simulink model "twist_filter_sl"  (R2018b)
settings: Solver=FixedStepDiscrete  StartTime=0.0  StopTime=inf  FixedStep=0.1  RelTol=1e-3
model workspace (MAT data in the model file):
  ERROR = 1e-08
undefined symbols (not defined in the file): Header, Twist
libraries: robotlib x5, simulink x1
settings Model: Creator=sdd  LastModifiedBy=sdd
settings DataIOCC: SaveOutput=off  SignalLogging=off  DSMLogging=off  SaveTime=off
settings OptimizationCC: EnhancedBackFolding=on  PassReuseOutputArgsThreshold=0  MaxStackSize=64  OptimizeBlockOrder=speed  DifferentSizesBufferReuse=on  OptimizationCustomize=off
settings DebuggingCC: ParameterTunabilityLossMsg=error  LibraryContextMissingDiagnostic=none
settings HardwareCC: ProdBitPerPointer=32  ProdBitPerSizeT=32  ProdBitPerPtrDiffT=32  ProdLargestAtomicFloat=None  ProdIntDivRoundTo=Undefined  ProdEndianess=Unspecified  ProdWordSize=32  ProdHWDeviceType=Generic->Unspecified (assume 32-bit Generic)  UseEmbeddedCoderFeatures=off
settings SFSimCC: SimUseLocalCustomCode=off  MATLABDynamicMemAlloc=off
settings RTWCC: SystemTargetFile=ert.tlc  HardwareBoard=Robot Operating System (ROS)  TLCOptions="-aInlineSetEventsForThisBaseRateFcn=TLC_FALSE -aSuppressMultiTaskScheduler=TLC_FALSE  -aRateBasedStepFcn=0"  TemplateMakefile=ert_default_tmf  GenerateReport=on  RTWUseLocalCustomCode=off  Toolchain=Catkin  LaunchReport=on  TargetLang=C++
settings CodeAppCC: ForceParamTrailComments=on  OperatorAnnotations=on
settings ERTTargetCC: ERTCustomFileBanners=off  SupportContinuousTime=on  SupportNonInlinedSFcns=on  RemoveResetFunc=off  ModelStepFunctionPrototypeControlCompliant=off

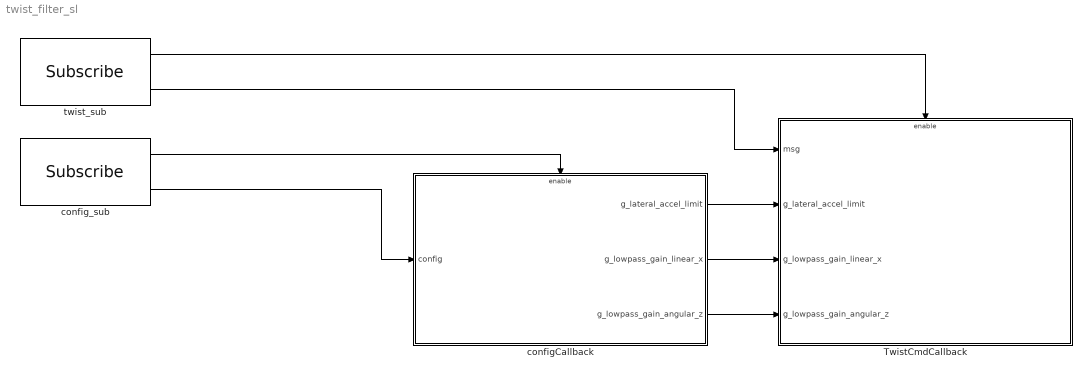
== system twist_filter_sl ==
  TwistCmdCallback : Subsystem
  configCallback : Subsystem
  config_sub : robotlib/Subscribe  topicSource=Select from ROS network  topic=/config/twist_filter  messageType=autoware_msgs/ConfigTwistFilter  sampleTime=-1  messageQueueLength=1
      settings: SourceProductBaseCode=RO
  twist_sub : robotlib/Subscribe  topicSource=Select from ROS network  topic=/twist_raw  messageType=geometry_msgs/TwistStamped  sampleTime=-1  messageQueueLength=1
      settings: SourceProductBaseCode=RO
  wires:
  configCallback/1(g_lateral_accel_limit) -> TwistCmdCallback/2(g_lateral_accel_limit)
  configCallback/2(g_lowpass_gain_linear_x) -> TwistCmdCallback/3(g_lowpass_gain_linear_x)
  configCallback/3(g_lowpass_gain_angular_z) -> TwistCmdCallback/4(g_lowpass_gain_angular_z)
  config_sub/1 -> configCallback/Enable
  config_sub/2 -> configCallback/1(config)
  twist_sub/1 -> TwistCmdCallback/Enable
  twist_sub/2 -> TwistCmdCallback/1(msg)

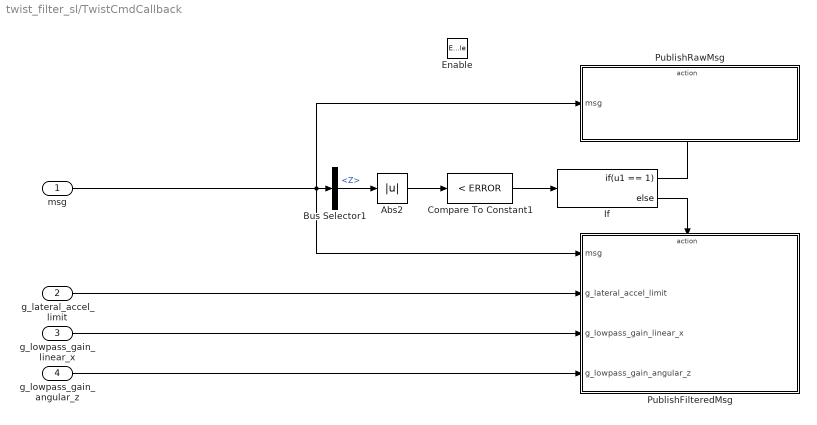
== system twist_filter_sl/TwistCmdCallback ==
  msg : Inport  Interpolate=off  BusOutputAsStruct=on
  g_lateral_accel_limit : Inport  Port=2
  g_lowpass_gain_linear_x : Inport  Port=3
  g_lowpass_gain_angular_z : Inport  Port=4
  Enable : EnablePort
  Abs2 : Abs
  Bus Selector1 : BusSelector  OutputSignals=Twist.Angular.Z
  Compare To Constant1 : simulink/Logic and Bit Operations/Compare To Constant  relop=<  const=ERROR  OutDataTypeStr=boolean
  If : If  IfExpression=u1 == 1
  PublishFilteredMsg : Subsystem
  PublishRawMsg : Subsystem  TreatAsAtomicUnit=on
  wires:
  g_lowpass_gain_angular_z/1 -> PublishFilteredMsg/4(g_lowpass_gain_angular_z)
  g_lowpass_gain_linear_x/1 -> PublishFilteredMsg/3(g_lowpass_gain_linear_x)
  Compare To Constant1/1 -> If/1
  If/2 -> PublishFilteredMsg/Action
  Bus Selector1/1 -> Abs2/1  "<Z>"
  msg/1 -> PublishFilteredMsg/1(msg), PublishRawMsg/1(msg), Bus Selector1/1
  Abs2/1 -> Compare To Constant1/1
  g_lateral_accel_limit/1 -> PublishFilteredMsg/2(g_lateral_accel_limit)
  If/1 -> PublishRawMsg/Action

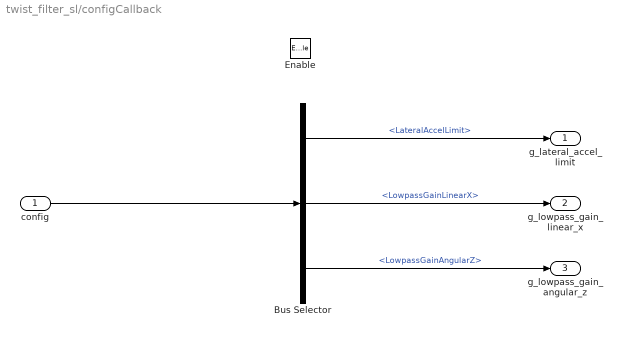
== system twist_filter_sl/configCallback ==
  config : Inport
  Enable : EnablePort
  Bus Selector : BusSelector  OutputSignals=LateralAccelLimit,LowpassGainLinearX,LowpassGainAngularZ
  g_lateral_accel_limit : Outport  InitialOutput=5
  g_lowpass_gain_linear_x : Outport  Port=2  InitialOutput=0
  g_lowpass_gain_angular_z : Outport  Port=3  InitialOutput=0
  wires:
  Bus Selector/3 -> g_lowpass_gain_angular_z/1  "<LowpassGainAngularZ>"
  Bus Selector/2 -> g_lowpass_gain_linear_x/1  "<LowpassGainLinearX>"
  config/1 -> Bus Selector/1
  Bus Selector/1 -> g_lateral_accel_limit/1  "<LateralAccelLimit>"

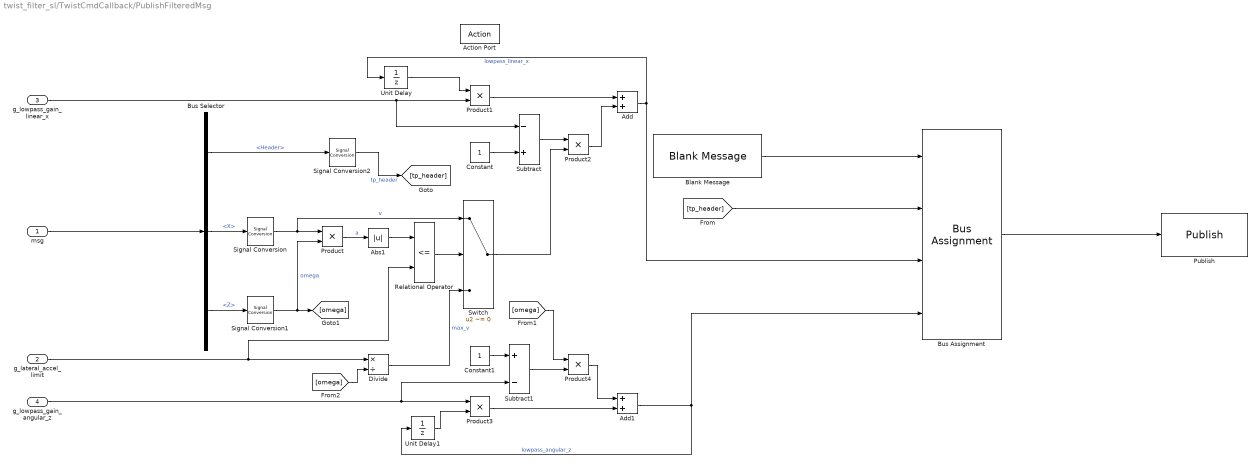
== system twist_filter_sl/TwistCmdCallback/PublishFilteredMsg ==
  msg : Inport
  g_lateral_accel_limit : Inport  Port=2
  g_lowpass_gain_linear_x : Inport  Port=3
  g_lowpass_gain_angular_z : Inport  Port=4
  Action Port : ActionPort  ActionType=else
  Abs1 : Abs
  Add : Sum
  Add1 : Sum
  Blank Message : robotlib/Blank Message  messageClass=Message  entityType=geometry_msgs/TwistStamped  messageType=geometry_msgs/TwistStamped  SampleTime=inf
      settings: SourceProductBaseCode=RO
  Bus Assignment : BusAssignment  AssignedSignals=Header,Twist.Linear.X,Twist.Angular.Z
  Bus Selector : BusSelector  OutputSignals=Header,Twist.Linear.X,Twist.Angular.Z
  Constant : Constant
  Constant1 : Constant
  Divide : Product  Inputs=*/
  Product{,1..4} (5 alike) : Product
  Publish : robotlib/Publish  topicSource=Specify your own  topic=/twist_cmd  messageType=geometry_msgs/TwistStamped  messageQueueLength=1
      settings: SourceProductBaseCode=RO
  Relational Operator : RelationalOperator  Operator=<=  OutDataTypeStr=boolean  RndMeth=Simplest
  Signal Conversion : SignalConversion  OverrideOpt=off
  Signal Conversion1 : SignalConversion  OverrideOpt=off
  Signal Conversion2 : SignalConversion  OverrideOpt=off
  Subtract : Sum  Inputs=-+
  Subtract1 : Sum  Inputs=+-
  Switch : Switch  Criteria=u2 ~= 0
  Unit Delay : UnitDelay  SampleTime=-1  StateName=lowpass_linear_x
  Unit Delay1 : UnitDelay  SampleTime=-1  StateName=lowpass_linear_x
  wires:
  Abs1/1 -> Relational Operator/1
  Unit Delay1/1 -> Product3/2
  Subtract/1 -> Product2/1
  Constant/1 -> Subtract/2
  Product1/1 -> Add/1
  Add/1 -> Bus Assignment/3, Unit Delay/1  "lowpass_linear_x"
  Divide/1 -> Switch/3  "max_v"
  g_lowpass_gain_linear_x/1 -> Subtract/1, Product1/2
  Product2/1 -> Add/2
  Subtract1/1 -> Product4/2
  Relational Operator/1 -> Switch/2
  Add1/1 -> Bus Assignment/4, Unit Delay1/1  "lowpass_angular_z"
  Switch/1 -> Product2/2
  g_lateral_accel_limit/1 -> Divide/1, Relational Operator/2
  g_lowpass_gain_angular_z/1 -> Product3/1, Subtract1/2
  Unit Delay/1 -> Product1/1
  Product3/1 -> Add1/2
  Signal Conversion1/1 -> [omega], Product/2  "omega"
  Constant1/1 -> Subtract1/1
  Product/1 -> Abs1/1  "a"
  Signal Conversion2/1 -> [tp_header]  "tp_header"
  Product4/1 -> Add1/1
  msg/1 -> Bus Selector/1
  Signal Conversion/1 -> Switch/1, Product/1  "v"
  Bus Selector/1 -> Signal Conversion2/1  "<Header>"
  Bus Selector/2 -> Signal Conversion/1  "<X>"
  Bus Selector/3 -> Signal Conversion1/1  "<Z>"
  [omega] -> Product4/1
  [omega] -> Divide/2
  Blank Message/1 -> Bus Assignment/1
  Bus Assignment/1 -> Publish/1
  [tp_header] -> Bus Assignment/2

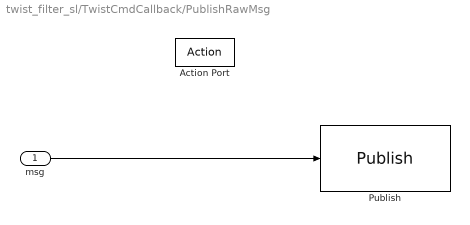
== system twist_filter_sl/TwistCmdCallback/PublishRawMsg ==
  msg : Inport
  Action Port : ActionPort  ActionType=then
  Publish : robotlib/Publish  topicSource=Specify your own  topic=/twist_cmd  messageType=geometry_msgs/TwistStamped  messageQueueLength=1
      settings: SourceProductBaseCode=RO
  wires:
  msg/1 -> Publish/1
